simulink model "APP_MyApplication"  (R2018b)
settings: Solver=VariableStepDiscrete  StartTime=0.0  StopTime=10  RelTol=1e-3
PreLoadFcn:
  | if(exist('MBDS_ModelCallback', 'file')), MBDS_ModelCallback('PreLoad'); end;
PostLoadFcn:
  | if(exist('MBDS_ModelCallback', 'file')), MBDS_ModelCallback('PostLoad'); end;
InitFcn:
  | if(exist('MBDS_ModelCallback', 'file')), MBDS_ModelCallback('Init'); end;
StartFcn:
  | if(exist('MBDS_ModelCallback', 'file')), MBDS_ModelCallback('Start'); end;
StopFcn:
  | if(exist('MBDS_ModelCallback', 'file')), MBDS_ModelCallback('Stop'); end;
undefined symbols (not defined in the file): sigbuilder_block, Ts
libraries: KIBES_Signal x499, simulink x8
(part 9 of 10)

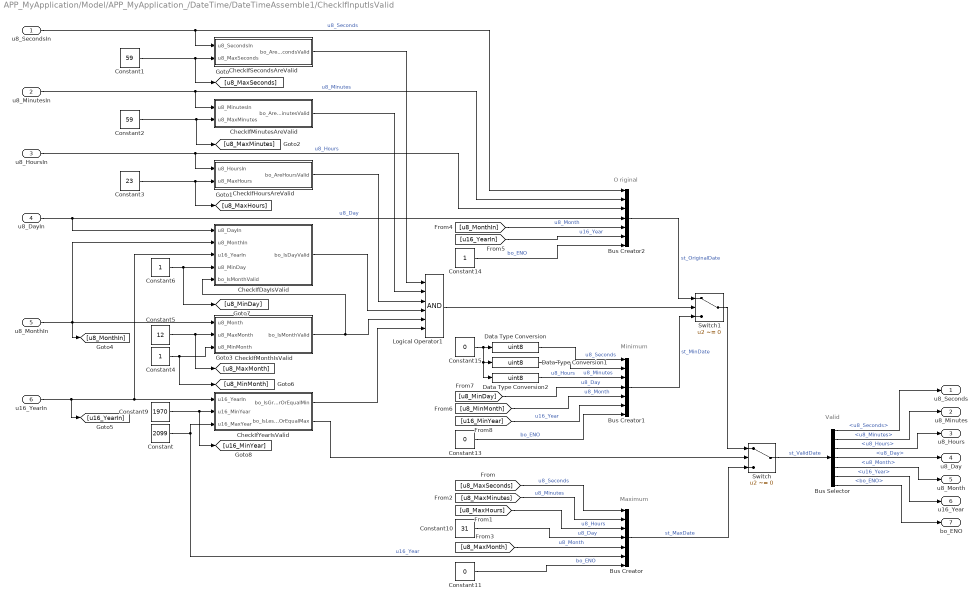
== system APP_MyApplication/Model/APP_MyApplication_/DateTime/DateTimeAssemble1/CheckIfInputIsValid ==
  note: Valid
  note: O riginal
  note: Minimum
  note: Maximum
  u8_SecondsIn : Inport  OutDataTypeStr=uint8
  u8_MinutesIn : Inport  Port=2  OutDataTypeStr=uint8
  u8_HoursIn : Inport  Port=3  OutDataTypeStr=uint8
  u8_DayIn : Inport  Port=4  OutDataTypeStr=uint8
  u8_MonthIn : Inport  Port=5  OutDataTypeStr=uint8
  u16_YearIn : Inport  Port=6  OutDataTypeStr=uint16
  Bus Creator : BusCreator  Inputs='u8_Seconds','u8_Minutes','u8_Hours','u8_Day','u8_Month','u16_Year','bo_ENO'
  Bus Creator1 : BusCreator  Inputs='u8_Seconds','u8_Minutes','u8_Hours','u8_Day','u8_Month','u16_Year','bo_ENO'
  Bus Creator2 : BusCreator  Inputs='u8_Seconds','u8_Minutes','u8_Hours','u8_Day','u8_Month','u16_Year','bo_ENO'
  Bus Selector : BusSelector  OutputSignals=u8_Seconds,u8_Minutes,u8_Hours,u8_Day,u8_Month,u16_Year,bo_ENO
  CheckIfDayIsValid : Subsystem
  CheckIfHoursAreValid : Subsystem
  CheckIfMinutesAreValid : Subsystem
  CheckIfMonthIsValid : Subsystem
  CheckIfSecondsAreValid : Subsystem
  CheckIfYearIsValid : Subsystem
  Constant : Constant  Value=2099  OutDataTypeStr=uint16
  Constant1 : Constant  Value=59  OutDataTypeStr=uint8
  Constant10 : Constant  Value=31  OutDataTypeStr=uint8
  Constant11 : Constant  Value=0  OutDataTypeStr=boolean
  Constant13 : Constant  Value=0  OutDataTypeStr=boolean
  Constant14 : Constant  OutDataTypeStr=boolean
  Constant15 : Constant  Value=0  OutDataTypeStr=uint8
  Constant2 : Constant  Value=59  OutDataTypeStr=uint8
  Constant3 : Constant  Value=23  OutDataTypeStr=uint8
  Constant4 : Constant  OutDataTypeStr=uint8
  Constant5 : Constant  Value=12  OutDataTypeStr=uint8
  Constant6 : Constant  OutDataTypeStr=uint8
  Constant9 : Constant  Value=1970  OutDataTypeStr=uint16
  Data Type Conversion : DataTypeConversion  OutDataTypeStr=uint8
  Data Type Conversion1 : DataTypeConversion  OutDataTypeStr=uint8
  Data Type Conversion2 : DataTypeConversion  OutDataTypeStr=uint8
  Logical Operator1 : Logic  Inputs=6  AllPortsSameDT=off  OutDataTypeStr=boolean
  Switch : Switch  Criteria=u2 ~= 0
  Switch1 : Switch  Criteria=u2 ~= 0
  u8_Seconds : Outport  OutDataTypeStr=uint8
  u8_Minutes : Outport  Port=2  OutDataTypeStr=uint8
  u8_Hours : Outport  Port=3  OutDataTypeStr=uint8
  u8_Day : Outport  Port=4  OutDataTypeStr=uint8
  u8_Month : Outport  Port=5  OutDataTypeStr=uint8
  u16_Year : Outport  Port=6  OutDataTypeStr=uint16
  bo_ENO : Outport  Port=7  OutDataTypeStr=boolean
  wires:
  u16_YearIn/1 -> CheckIfYearIsValid/1(u16_YearIn), CheckIfDayIsValid/3(u16_YearIn), [u16_YearIn]
  Constant/1 -> Bus Creator/6, CheckIfYearIsValid/3(u16_MaxYear)  "u16_Year"
  u8_HoursIn/1 -> Bus Creator2/3, CheckIfHoursAreValid/1(u8_HoursIn)  "u8_Hours"
  u8_MinutesIn/1 -> Bus Creator2/2, CheckIfMinutesAreValid/1(u8_MinutesIn)  "u8_Minutes"
  u8_SecondsIn/1 -> CheckIfSecondsAreValid/1(u8_SecondsIn), Bus Creator2/1  "u8_Seconds"
  u8_DayIn/1 -> Bus Creator2/4, CheckIfDayIsValid/1(u8_DayIn)  "u8_Day"
  Constant5/1 -> CheckIfMonthIsValid/2(u8_MaxMonth), [u8_MaxMonth]
  CheckIfMinutesAreValid/1(bo_AreMinutesValid) -> Logical Operator1/2
  CheckIfHoursAreValid/1(bo_AreHoursValid) -> Logical Operator1/3
  Constant9/1 -> [u16_MinYear], CheckIfYearIsValid/2(u16_MinYear)
  Constant11/1 -> Bus Creator/7  "bo_ENO"
  [u8_MaxMinutes] -> Bus Creator/2  "u8_Minutes"
  [u8_MaxHours] -> Bus Creator/3  "u8_Hours"
  Constant3/1 -> CheckIfHoursAreValid/2(u8_MaxHours), [u8_MaxHours]
  Constant10/1 -> Bus Creator/4  "u8_Day"
  [u8_MaxMonth] -> Bus Creator/5  "u8_Month"
  [u8_MinMonth] -> Bus Creator1/5  "u8_Month"
  Logical Operator1/1 -> Switch1/2
  Bus Creator1/1 -> Switch1/3  "st_MinDate"
  [u8_MonthIn] -> Bus Creator2/5  "u8_Month"
  [u16_YearIn] -> Bus Creator2/6  "u16_Year"
  Constant13/1 -> Bus Creator1/7  "bo_ENO"
  Bus Selector/4 -> u8_Day/1  "<u8_Day>"
  Bus Selector/3 -> u8_Hours/1  "<u8_Hours>"
  Bus Selector/2 -> u8_Minutes/1  "<u8_Minutes>"
  Bus Selector/1 -> u8_Seconds/1  "<u8_Seconds>"
  Bus Selector/6 -> u16_Year/1  "<u16_Year>"
  Bus Selector/7 -> bo_ENO/1  "<bo_ENO>"
  Bus Creator2/1 -> Switch1/1  "st_OriginalDate"
  Switch1/1 -> Switch/1
  Bus Creator/1 -> Switch/3  "st_MaxDate"
  Switch/1 -> Bus Selector/1  "st_ValidDate"
  Constant14/1 -> Bus Creator2/7  "bo_ENO"
  Data Type Conversion/1 -> Bus Creator1/1  "u8_Seconds"
  [u8_MinDay] -> Bus Creator1/4  "u8_Day"
  Constant15/1 -> Data Type Conversion2/1, Data Type Conversion1/1, Data Type Conversion/1
  [u8_MaxSeconds] -> Bus Creator/1  "u8_Seconds"
  Bus Selector/5 -> u8_Month/1  "<u8_Month>"
  u8_MonthIn/1 -> CheckIfDayIsValid/2(u8_MonthIn), [u8_MonthIn], CheckIfMonthIsValid/1(u8_Month)
  CheckIfDayIsValid/1(bo_IsDayValid) -> Logical Operator1/4
  Constant1/1 -> [u8_MaxSeconds], CheckIfSecondsAreValid/2(u8_MaxSeconds)
  CheckIfSecondsAreValid/1(bo_AreSecondsValid) -> Logical Operator1/1
  Constant2/1 -> [u8_MaxMinutes], CheckIfMinutesAreValid/2(u8_MaxMinutes)
  CheckIfMonthIsValid/1(bo_IsMonthValid) -> CheckIfDayIsValid/5(bo_IsMonthValid), Logical Operator1/5
  CheckIfYearIsValid/1(bo_IsGreaterOrEqualMin) -> Logical Operator1/6
  CheckIfYearIsValid/2(bo_IsLessOrEqualMax) -> Switch/2
  Constant4/1 -> [u8_MinMonth], CheckIfMonthIsValid/3(u8_MinMonth)
  Constant6/1 -> [u8_MinDay], CheckIfDayIsValid/4(u8_MinDay)
  [u16_MinYear] -> Bus Creator1/6  "u16_Year"
  Data Type Conversion1/1 -> Bus Creator1/2  "u8_Minutes"
  Data Type Conversion2/1 -> Bus Creator1/3  "u8_Hours"

== system APP_MyApplication/Model/APP_MyApplication_/DateTime/DateTimeAssemble1/ConvertToDateTime ==
  u8_Seconds : Inport  OutDataTypeStr=uint8
  u8_Minutes : Inport  Port=2  OutDataTypeStr=uint8
  u8_Hours : Inport  Port=3  OutDataTypeStr=uint8
  u16_NrOfDays : Inport  Port=4  OutDataTypeStr=uint16
  Add : Sum  Inputs=++++  OutDataTypeStr=uint32
  ConvertDaysToSeconds : Subsystem
  ConvertHoursToSeconds : Subsystem
  ConvertMinutesToSeconds : Subsystem
  u32_DateTime : Outport  OutDataTypeStr=uint32
  wires:
  u8_Seconds/1 -> Add/1
  Add/1 -> u32_DateTime/1
  ConvertMinutesToSeconds/1(u16_SecFromMins) -> Add/2
  ConvertHoursToSeconds/1(u32_SecFromHrs) -> Add/3
  ConvertDaysToSeconds/1(u32_SecFromDays) -> Add/4
  u8_Minutes/1 -> ConvertMinutesToSeconds/1(u8_Minutes)
  u8_Hours/1 -> ConvertHoursToSeconds/1(u8_Hours)
  u16_NrOfDays/1 -> ConvertDaysToSeconds/1(u16_NrOfDays)

== system APP_MyApplication/Model/APP_MyApplication_/DateTime/DateTimeAssemble1/ConvertToNrOfDays ==
  note: Convert to number of days
  u8_Day : Inport  OutDataTypeStr=uint8
  u8_Month : Inport  Port=2  OutDataTypeStr=uint8
  u16_Year : Inport  Port=3  OutDataTypeStr=uint16
  AddDays : Subsystem
  AddDaysForCompleteMonths : Subsystem  TreatAsAtomicUnit=on
  AddDaysForCompleteYears : Subsystem
  CheckIfDateInLeapYearBeforeMarch : Subsystem
  Subtract2 : Sum  Inputs=+++-  OutDataTypeStr=uint16
  u16_NrOfDays : Outport  OutDataTypeStr=uint16
  wires:
  u16_Year/1 -> CheckIfDateInLeapYearBeforeMarch/2(u16_Year), AddDaysForCompleteYears/1(u16_Year)
  Subtract2/1 -> u16_NrOfDays/1
  u8_Month/1 -> CheckIfDateInLeapYearBeforeMarch/1(u8_Month), AddDaysForCompleteMonths/1(u8_Month)
  u8_Day/1 -> AddDays/1(u8_Day)
  AddDaysForCompleteMonths/1(u16_DaysForMonths) -> Subtract2/2
  AddDays/1(u8_CompleteDays) -> Subtract2/1
  AddDaysForCompleteYears/1(u16_DaysForYears) -> Subtract2/3
  CheckIfDateInLeapYearBeforeMarch/1(bo_MinusOne) -> Subtract2/4

== system APP_MyApplication/Model/APP_MyApplication_/DateTime/DateTimeDisassemble/CheckIfTimeDataIsValid ==
  note: 2099-12-31-23:59:59
  note: Check if time data is valid
  u32_DateTime : Inport  OutDataTypeStr=uint32
  Constant14 : Constant  Value=4102444799  OutDataTypeStr=uint32
  Relational Operator : RelationalOperator  Operator=<=  OutDataTypeStr=boolean  RndMeth=Nearest
  bo_ENO : Outport  OutDataTypeStr=boolean
  wires:
  Constant14/1 -> Relational Operator/2
  u32_DateTime/1 -> Relational Operator/1
  Relational Operator/1 -> bo_ENO/1

== system APP_MyApplication/Model/APP_MyApplication_/DateTime/DateTimeDisassemble/CheckLeapYearsAndRemainingDays ==
  note: Year
  note: Check leap year and calculate remaining days in current year
  note: avoid overflow
  u16_NrOfDays : Inport  OutDataTypeStr=uint16
  Add3 : Sum  Inputs=++-  OutDataTypeStr=uint16
  CalculateLeapYearsSince1970 : Subsystem
  CalculateRemainingDays : Subsystem
  CheckIfCorrectedTempYearIsLeap : Subsystem
  CheckIfTempYearIsCorrect : Subsystem
  CheckLeapYear : Subsystem
  Constant2 : Constant  OutDataTypeStr=uint16
  Constant6 : Constant  Value=0  OutDataTypeStr=uint16
  DaysPerNonLeapYear : Constant  Value=365  OutDataTypeStr=uint16
  Math Function3 : Math  Operator=rem  OutputSignalType=real  SaturateOnIntegerOverflow=on
  Relational Operator1 : RelationalOperator  Operator===  OutDataTypeStr=boolean  RndMeth=Nearest  InputSameDT=on
  Switch1 : Switch  Criteria=u2 ~= 0  OutDataTypeStr=uint16
  u16_TempDate : Outport  OutDataTypeStr=uint16
  u16_Year : Outport  Port=2  OutDataTypeStr=uint16
  bo_LeapYear : Outport  Port=3  OutDataTypeStr=boolean
  wires:
  u16_NrOfDays/1 -> CalculateLeapYearsSince1970/1(u16_NrOfDays), Math Function3/1
  DaysPerNonLeapYear/1 -> CalculateRemainingDays/5(u16_DaysPerCommonYear), Math Function3/2, CalculateLeapYearsSince1970/2(u16_DaysPerCommonYear)
  Math Function3/1 -> CalculateRemainingDays/3(u16_TempRemainingDays), CheckIfTempYearIsCorrect/1(u16_TempRemainingDays)
  Switch1/1 -> CheckLeapYear/1(u16_Year), u16_Year/1
  CalculateLeapYearsSince1970/2(u16_TempYear) -> Switch1/1, Add3/2, Relational Operator1/2
  Add3/1 -> Switch1/3, CheckIfCorrectedTempYearIsLeap/1(u16_CorrectedTempYear)
  CheckLeapYear/1(bo_LeapYear) -> bo_LeapYear/1
  Constant6/1 -> Relational Operator1/1
  Constant2/1 -> Add3/3
  Relational Operator1/1 -> Add3/1
  CalculateLeapYearsSince1970/1(u16_NrOfLeapYears) -> [u16_NrOfLeapYears]
  [u16_NrOfLeapYears] -> CheckIfTempYearIsCorrect/2(u16_NrOfLeapYears)
  CheckIfTempYearIsCorrect/1(bo_IsTempYearCorrect) -> Switch1/2, CalculateRemainingDays/2(bo_IsTempYearCorrect)
  CalculateRemainingDays/1(u16_TempDate) -> u16_TempDate/1
  CheckIfCorrectedTempYearIsLeap/1(bo_IsCorrectedYearLeapYear) -> CalculateRemainingDays/1(bo_IsCorrectedYearLeapYear)
  [u16_NrOfLeapYears] -> CalculateRemainingDays/4(u16_NrOfLeapYears)

== system APP_MyApplication/Model/APP_MyApplication_/DateTime/DateTimeDisassemble/ConvertToDayOfWeek ==
  note: 1970-01-01 is Thursday
  note: Convert to day of week
  u16_NrOfDays : Inport  OutDataTypeStr=uint16
  Add2 : Sum  OutDataTypeStr=uint16
  Add3 : Sum  OutDataTypeStr=uint16
  Constant3 : Constant  Value=7  OutDataTypeStr=uint16
  Constant4 : Constant  Value=3  OutDataTypeStr=uint8
  Constant5 : Constant  OutDataTypeStr=uint8
  Data Type Conversion3 : DataTypeConversion  OutDataTypeStr=uint8
  Math Function : Math  Operator=rem  OutputSignalType=real  SaturateOnIntegerOverflow=on
  u8_DayOfWeek : Outport  OutDataTypeStr=uint8
  wires:
  Data Type Conversion3/1 -> u8_DayOfWeek/1
  Constant5/1 -> Add3/2
  Constant3/1 -> Math Function/2
  Constant4/1 -> Add2/2
  Add2/1 -> Math Function/1
  Math Function/1 -> Add3/1
  Add3/1 -> Data Type Conversion3/1
  u16_NrOfDays/1 -> Add2/1

== system APP_MyApplication/Model/APP_MyApplication_/DateTime/DateTimeDisassemble/ConvertToMonthAndDay ==
  note: Days per month
  note: Count number of cycles (= Month - 1)
  note: Check if there are less days remaining than the next month has
  note: Convert to month and day
  u16_TempDate : Inport  OutDataTypeStr=uint16
  bo_LeapYear : Inport  Port=2  OutDataTypeStr=boolean
  Add5 : Sum  OutDataTypeStr=uint8
  CheckNrOfDaysInNextMonth : Subsystem
  Constant1 : Constant  Value=[0 31 28 31 30 31 30 31 31 30 31 30 31]  OutDataTypeStr=uint8
  Data Type Conversion : DataTypeConversion  OutDataTypeStr=uint8
  Data Type Conversion1 : DataTypeConversion  OutDataTypeStr=uint16
  Relational Operator1 : RelationalOperator  OutDataTypeStr=boolean  RndMeth=Nearest  InputSameDT=on
  SubstractDaysOfMonths : Subsystem
  Unit Delay1 : UnitDelay  SampleTime=-1
  While Iterator : WhileIterator  MaxIters=12  WhileBlockType=do-while  ResetStates=reset  ShowIterationPort=on  OutputDataType=int8
  u8_MonthMinusOne : Outport  OutDataTypeStr=uint8
  u16_DayMinusOne : Outport  Port=2  OutDataTypeStr=uint16
  wires:
  bo_LeapYear/1 -> SubstractDaysOfMonths/2(bo_LeapYear), CheckNrOfDaysInNextMonth/3(bo_LeapYear)
  Relational Operator1/1 -> Data Type Conversion/1, While Iterator/1
  While Iterator/1 -> SubstractDaysOfMonths/3(i8_IterationNr), CheckNrOfDaysInNextMonth/2(i8_IterationNr)
  Add5/1 -> u8_MonthMinusOne/1, Unit Delay1/1
  Unit Delay1/1 -> Add5/2
  Data Type Conversion/1 -> Add5/1
  SubstractDaysOfMonths/1(u16_RemainingDays) -> u16_DayMinusOne/1, Relational Operator1/1
  CheckNrOfDaysInNextMonth/1(u8_DaysInNextMonth) -> Data Type Conversion1/1
  u16_TempDate/1 -> SubstractDaysOfMonths/1(u16_TempDate)
  Constant1/1 -> SubstractDaysOfMonths/4(u8_DaysPerMonth), CheckNrOfDaysInNextMonth/1(u8_DaysPerMonth)
  Data Type Conversion1/1 -> Relational Operator1/2

== system APP_MyApplication/Model/APP_MyApplication_/DateTime/DateTimeDisassemble/ConvertToTimeAndNrOfDays ==
  note: Convert date time to time and number of days
  u32_DateTime : Inport  OutDataTypeStr=uint32
  CalculateHours : Subsystem
  CalculateMinutes : Subsystem
  CalculateSeconds : Subsystem
  u8_Seconds : Outport  OutDataTypeStr=uint8
  u8_Minutes : Outport  Port=2  OutDataTypeStr=uint8
  u8_Hours : Outport  Port=3  OutDataTypeStr=uint8
  u16_NrOfDays : Outport  Port=4  OutDataTypeStr=uint16
  wires:
  CalculateSeconds/1(u8_Seconds) -> u8_Seconds/1
  CalculateHours/2(u16_NrOfDays) -> u16_NrOfDays/1
  u32_DateTime/1 -> CalculateSeconds/1(u32_TimeInSeconds)
  CalculateSeconds/2(u32_TempDateMin) -> CalculateMinutes/1(u32_TempDateMin)
  CalculateMinutes/1(u8_Minutes) -> u8_Minutes/1
  CalculateMinutes/2(u32_TempDateHrs) -> CalculateHours/1(u32_TempDateHrs)
  CalculateHours/1(u8_Hours) -> u8_Hours/1

== system APP_MyApplication/Model/APP_MyApplication_/EEProm/TimerPulse/EdgeRising ==
  note: EdgeRising
  u : Inport  OutDataTypeStr=boolean
  Data Type Duplicate : DataTypeDuplicate
  IV : Constant  Value=0  OutDataTypeStr=Inherit: Inherit via back propagation
  NoReset : Subsystem
  R : Constant  Value=0  OutDataTypeStr=boolean
  Relational Operator : RelationalOperator  Operator=<  OutDataTypeStr=boolean  RndMeth=Nearest  InputSameDT=on
  Unit Delay : UnitDelay  SampleTime=-1
  y : Outport
  wires:
  IV/1 -> NoReset/1(Unused1), Data Type Duplicate/2
  u/1 -> Unit Delay/1, Relational Operator/2, Data Type Duplicate/1
  R/1 -> NoReset/2(Unused2)
  NoReset/1(y) -> Relational Operator/1
  Unit Delay/1 -> NoReset/3(u)
  Relational Operator/1 -> y/1

== system APP_MyApplication/Model/APP_MyApplication_/EEProm/TimerPulse/TimeSource ==
  note: TimeSource
  Constant : Constant  Value=Value  OutDataTypeStr=uint32  LockScale=on
  Out : Outport
  wires:
  Constant/1 -> Out/1

== system APP_MyApplication/Model/APP_MyApplication_/EEProm/TimerPulse/Timer_RE1 ==
  note: Timer_RE
  R : Inport  OutDataTypeStr=boolean
  IV : Inport  Port=2
  Constant : Constant  Value=0  OutDataTypeStr=Inherit: Inherit via back propagation
  Constant1 : Constant  Value=0  OutDataTypeStr=Inherit: Inherit via back propagation
  Constant2 : Constant  Value=0  OutDataTypeStr=Inherit: Inherit via back propagation
  Data Type Duplicate : DataTypeDuplicate  NumInputPorts=3
  DoubleReset : Subsystem
  E : Constant  OutDataTypeStr=boolean
  NoEnable : Subsystem
  Relational Operator : RelationalOperator  Operator=<=  OutDataTypeStr=boolean  RndMeth=Nearest
  Relational Operator1 : RelationalOperator  Operator=>  OutDataTypeStr=boolean  RndMeth=Nearest
  Relational Operator2 : RelationalOperator  Operator=>  OutDataTypeStr=boolean  RndMeth=Nearest  InputSameDT=on
  Subtract : Sum  Inputs=+-  OutDataTypeStr=Inherit: Inherit via back propagation
  Switch1 : Switch  Criteria=u2 ~= 0  OutDataTypeStr=Inherit: Inherit via back propagation
  Unit Delay : UnitDelay  SampleTime=-1
  dT : Constant  Value=1000*Ts  OutDataTypeStr=Inherit: Inherit via back propagation
  x : Terminator
  y : Outport
  wires:
  R/1 -> DoubleReset/2(R1)
  E/1 -> NoEnable/2(Unused1)
  IV/1 -> Data Type Duplicate/1, DoubleReset/1(IV)
  Relational Operator/1 -> DoubleReset/3(R2)
  DoubleReset/1(y) -> Relational Operator2/1, Unit Delay/1, x/1, Data Type Duplicate/3
  Constant2/1 -> Relational Operator2/2
  Constant/1 -> Switch1/3
  Subtract/1 -> Switch1/1
  Relational Operator1/1 -> Switch1/2
  Switch1/1 -> NoEnable/1(u)
  dT/1 -> Subtract/2, Relational Operator1/2
  Unit Delay/1 -> NoEnable/3(Unused2), Relational Operator1/1, Subtract/1, Relational Operator/1, Data Type Duplicate/2
  Constant1/1 -> Relational Operator/2
  NoEnable/1(y) -> DoubleReset/4(u)
  Relational Operator2/1 -> y/1

== system APP_MyApplication/Model/APP_MyApplication_/EEProm/TimerPulse1/EdgeRising ==
  note: EdgeRising
  u : Inport  OutDataTypeStr=boolean
  Data Type Duplicate : DataTypeDuplicate
  IV : Constant  Value=0  OutDataTypeStr=Inherit: Inherit via back propagation
  NoReset : Subsystem
  R : Constant  Value=0  OutDataTypeStr=boolean
  Relational Operator : RelationalOperator  Operator=<  OutDataTypeStr=boolean  RndMeth=Nearest  InputSameDT=on
  Unit Delay : UnitDelay  SampleTime=-1
  y : Outport
  wires:
  IV/1 -> NoReset/1(Unused1), Data Type Duplicate/2
  u/1 -> Unit Delay/1, Relational Operator/2, Data Type Duplicate/1
  R/1 -> NoReset/2(Unused2)
  NoReset/1(y) -> Relational Operator/1
  Unit Delay/1 -> NoReset/3(u)
  Relational Operator/1 -> y/1

== system APP_MyApplication/Model/APP_MyApplication_/EEProm/TimerPulse1/TimeSource ==
  note: TimeSource
  Constant : Constant  Value=Value  OutDataTypeStr=uint32  LockScale=on
  Out : Outport
  wires:
  Constant/1 -> Out/1

== system APP_MyApplication/Model/APP_MyApplication_/EEProm/TimerPulse1/Timer_RE1 ==
  note: Timer_RE
  R : Inport  OutDataTypeStr=boolean
  IV : Inport  Port=2
  Constant : Constant  Value=0  OutDataTypeStr=Inherit: Inherit via back propagation
  Constant1 : Constant  Value=0  OutDataTypeStr=Inherit: Inherit via back propagation
  Constant2 : Constant  Value=0  OutDataTypeStr=Inherit: Inherit via back propagation
  Data Type Duplicate : DataTypeDuplicate  NumInputPorts=3
  DoubleReset : Subsystem
  E : Constant  OutDataTypeStr=boolean
  NoEnable : Subsystem
  Relational Operator : RelationalOperator  Operator=<=  OutDataTypeStr=boolean  RndMeth=Nearest
  Relational Operator1 : RelationalOperator  Operator=>  OutDataTypeStr=boolean  RndMeth=Nearest
  Relational Operator2 : RelationalOperator  Operator=>  OutDataTypeStr=boolean  RndMeth=Nearest  InputSameDT=on
  Subtract : Sum  Inputs=+-  OutDataTypeStr=Inherit: Inherit via back propagation
  Switch1 : Switch  Criteria=u2 ~= 0  OutDataTypeStr=Inherit: Inherit via back propagation
  Unit Delay : UnitDelay  SampleTime=-1
  dT : Constant  Value=1000*Ts  OutDataTypeStr=Inherit: Inherit via back propagation
  x : Terminator
  y : Outport
  wires:
  R/1 -> DoubleReset/2(R1)
  E/1 -> NoEnable/2(Unused1)
  IV/1 -> Data Type Duplicate/1, DoubleReset/1(IV)
  Relational Operator/1 -> DoubleReset/3(R2)
  DoubleReset/1(y) -> Relational Operator2/1, Unit Delay/1, x/1, Data Type Duplicate/3
  Constant2/1 -> Relational Operator2/2
  Constant/1 -> Switch1/3
  Subtract/1 -> Switch1/1
  Relational Operator1/1 -> Switch1/2
  Switch1/1 -> NoEnable/1(u)
  dT/1 -> Subtract/2, Relational Operator1/2
  Unit Delay/1 -> NoEnable/3(Unused2), Relational Operator1/1, Subtract/1, Relational Operator/1, Data Type Duplicate/2
  Constant1/1 -> Relational Operator/2
  NoEnable/1(y) -> DoubleReset/4(u)
  Relational Operator2/1 -> y/1

== system APP_MyApplication/Model/APP_MyApplication_/TimerPulse/EdgeRising/NoReset ==
  Unused1 : Inport
  Unused2 : Inport  Port=2
  u : Inport  Port=3
  Terminator : Terminator
  Terminator1 : Terminator
  y : Outport
  wires:
  u/1 -> y/1
  Unused1/1 -> Terminator1/1
  Unused2/1 -> Terminator/1

== system APP_MyApplication/Model/APP_MyApplication_/TimerPulse/Timer_RE1/DoubleReset ==
  IV : Inport
  R1 : Inport  Port=2
  R2 : Inport  Port=3
  u : Inport  Port=4
  Logical Operator : Logic  AllPortsSameDT=off  OutDataTypeStr=boolean
  Switch1 : Switch  Criteria=u2 ~= 0  OutDataTypeStr=Inherit: Inherit via back propagation  InputSameDT=on
  y : Outport
  wires:
  u/1 -> Switch1/3
  Switch1/1 -> y/1
  IV/1 -> Switch1/1
  Logical Operator/1 -> Switch1/2
  R1/1 -> Logical Operator/1
  R2/1 -> Logical Operator/2

== system APP_MyApplication/Model/APP_MyApplication_/TimerPulse/Timer_RE1/NoEnable ==
  u : Inport
  Unused1 : Inport  Port=2
  Unused2 : Inport  Port=3
  Terminator : Terminator
  Terminator1 : Terminator
  y : Outport
  wires:
  Unused2/1 -> Terminator1/1
  u/1 -> y/1
  Unused1/1 -> Terminator/1

== system APP_MyApplication/Model/APP_MyApplication_/DTC/DateTimeDisassemble/CheckLeapYearsAndRemainingDays/CalculateLeapYearsSince1970 ==
  u16_NrOfDays : Inport  OutDataTypeStr=uint16
  u16_DaysPerCommonYear : Inport  Port=2  OutDataTypeStr=uint16
  Add : Sum  OutDataTypeStr=uint16
  Constant : Constant  OutDataTypeStr=uint16
  Constant1 : Constant  Value=4  OutDataTypeStr=uint16
  Divide : Product  Inputs=*/  OutDataTypeStr=uint16
  Divide1 : Product  Inputs=*/  OutDataTypeStr=uint16
  u16_NrOfLeapYears : Outport  OutDataTypeStr=uint16
  u16_TempYear : Outport  Port=2  OutDataTypeStr=uint16
  wires:
  Divide/1 -> Add/1, u16_TempYear/1
  Constant/1 -> Add/2
  Constant1/1 -> Divide1/2
  Add/1 -> Divide1/1
  Divide1/1 -> u16_NrOfLeapYears/1
  u16_NrOfDays/1 -> Divide/1
  u16_DaysPerCommonYear/1 -> Divide/2

== system APP_MyApplication/Model/APP_MyApplication_/DTC/DateTimeDisassemble/CheckLeapYearsAndRemainingDays/CalculateRemainingDays ==
  bo_IsCorrectedYearLeapYear : Inport  OutDataTypeStr=boolean
  bo_IsTempYearCorrect : Inport  Port=2  OutDataTypeStr=boolean
  u16_TempRemainingDays : Inport  Port=3  OutDataTypeStr=uint16
  u16_NrOfLeapYears : Inport  Port=4  OutDataTypeStr=uint16
  u16_DaysPerCommonYear : Inport  Port=5  OutDataTypeStr=uint16
  Add : Sum  OutDataTypeStr=uint16
  Add1 : Sum  Inputs=++-  OutDataTypeStr=uint16
  Constant : Constant  OutDataTypeStr=uint16
  Subtract : Sum  Inputs=+-  OutDataTypeStr=uint16  SaturateOnIntegerOverflow=on
      settings: AttributesFormatString=Saturate: %<SaturateOnIntegerOverflow>
  Switch : Switch  Criteria=u2 ~= 0  OutDataTypeStr=uint16
  Switch1 : Switch  Criteria=u2 ~= 0  OutDataTypeStr=uint16
  u16_TempDate : Outport  OutDataTypeStr=uint16
  wires:
  u16_TempRemainingDays/1 -> Add1/1, Subtract/1
  u16_NrOfLeapYears/1 -> Add1/3, Subtract/2
  u16_DaysPerCommonYear/1 -> Add1/2
  Constant/1 -> Add/1
  bo_IsCorrectedYearLeapYear/1 -> Switch1/2
  Add1/1 -> Add/2, Switch1/3
  Add/1 -> Switch1/1
  Switch1/1 -> Switch/3
  Switch/1 -> u16_TempDate/1
  bo_IsTempYearCorrect/1 -> Switch/2
  Subtract/1 -> Switch/1

== system APP_MyApplication/Model/APP_MyApplication_/DTC/DateTimeDisassemble/CheckLeapYearsAndRemainingDays/CheckIfCorrectedTempYearIsLeap ==
  u16_CorrectedTempYear : Inport  OutDataTypeStr=uint16
  Add : Sum  OutDataTypeStr=uint16
  Constant : Constant  Value=2  OutDataTypeStr=uint16
  Constant1 : Constant  Value=4  OutDataTypeStr=uint16
  Constant2 : Constant  Value=0  OutDataTypeStr=uint16
  Math Function : Math  Operator=rem  OutputSignalType=real  SaturateOnIntegerOverflow=on
  Relational Operator : RelationalOperator  Operator===  OutDataTypeStr=boolean  RndMeth=Nearest
  bo_IsCorrectedYearLeapYear : Outport  OutDataTypeStr=boolean
  wires:
  u16_CorrectedTempYear/1 -> Add/1
  Add/1 -> Math Function/1
  Math Function/1 -> Relational Operator/1
  Constant/1 -> Add/2
  Constant1/1 -> Math Function/2
  Constant2/1 -> Relational Operator/2
  Relational Operator/1 -> bo_IsCorrectedYearLeapYear/1

== system APP_MyApplication/Model/APP_MyApplication_/DTC/DateTimeDisassemble/CheckLeapYearsAndRemainingDays/CheckIfTempYearIsCorrect ==
  u16_TempRemainingDays : Inport  OutDataTypeStr=uint16
  u16_NrOfLeapYears : Inport  Port=2  OutDataTypeStr=uint16
  Relational Operator : RelationalOperator  OutDataTypeStr=boolean  RndMeth=Nearest
  bo_IsTempYearCorrect : Outport  OutDataTypeStr=boolean
  wires:
  u16_TempRemainingDays/1 -> Relational Operator/1
  u16_NrOfLeapYears/1 -> Relational Operator/2
  Relational Operator/1 -> bo_IsTempYearCorrect/1

== system APP_MyApplication/Model/APP_MyApplication_/DTC/DateTimeDisassemble/CheckLeapYearsAndRemainingDays/CheckLeapYear ==
  note: check if the current year is a leap year
  u16_Year : Inport  OutDataTypeStr=uint16
  Add6 : Sum  OutDataTypeStr=uint16
  Constant : Constant  Value=2  OutDataTypeStr=uint8
  Constant1 : Constant  Value=4  OutDataTypeStr=uint16
  Constant9 : Constant  Value=0  OutDataTypeStr=uint16
  Math Function : Math  Operator=rem  OutputSignalType=real  SaturateOnIntegerOverflow=on
  Relational Operator2 : RelationalOperator  Operator===  OutDataTypeStr=boolean  RndMeth=Nearest  InputSameDT=on
  bo_LeapYear : Outport  OutDataTypeStr=boolean
  wires:
  Add6/1 -> Math Function/1
  Relational Operator2/1 -> bo_LeapYear/1
  u16_Year/1 -> Add6/1
  Math Function/1 -> Relational Operator2/1
  Constant9/1 -> Relational Operator2/2
  Constant/1 -> Add6/2
  Constant1/1 -> Math Function/2

== system APP_MyApplication/Model/APP_MyApplication_/DTC/DateTimeDisassemble/ConvertToMonthAndDay/CheckNrOfDaysInNextMonth ==
  u8_DaysPerMonth : Inport  OutDataTypeStr=uint8
  i8_IterationNr : Inport  Port=2  OutDataTypeStr=int8
  bo_LeapYear : Inport  Port=3  OutDataTypeStr=boolean
  Add1 : Sum  OutDataTypeStr=uint8
  CheckNextMonthFebLeapYear : Subsystem
  Selector : Selector  IndexMode=Zero-based  InputPortWidth=13  IndexOptions=Index vector (port)  Indices=[1 3]  OutputSizes=1
  u8_DaysInNextMonth : Outport  OutDataTypeStr=uint8
  wires:
  bo_LeapYear/1 -> CheckNextMonthFebLeapYear/2(bo_LeapYear)
  i8_IterationNr/1 -> Selector/2, CheckNextMonthFebLeapYear/1(i8_IterationNr)
  u8_DaysPerMonth/1 -> Selector/1
  Selector/1 -> Add1/1
  CheckNextMonthFebLeapYear/1(bo_IsNextFebLeapYear) -> Add1/2
  Add1/1 -> u8_DaysInNextMonth/1

== system APP_MyApplication/Model/APP_MyApplication_/DTC/DateTimeDisassemble/ConvertToMonthAndDay/SubstractDaysOfMonths ==
  u16_TempDate : Inport  OutDataTypeStr=uint16
  bo_LeapYear : Inport  Port=2  OutDataTypeStr=boolean
  i8_IterationNr : Inport  Port=3  OutDataTypeStr=int8
  u8_DaysPerMonth : Inport  Port=4  OutDataTypeStr=uint8
  Add : Sum  OutDataTypeStr=uint16
  Add1 : Sum  OutDataTypeStr=uint16
  Add2 : Sum  Inputs=+-  OutDataTypeStr=uint8
  CheckCurrMonthFebLeapYear : Subsystem
  Constant : Constant  OutDataTypeStr=int8
  Selector : Selector  IndexMode=Zero-based  InputPortWidth=13  IndexOptions=Index vector (port)  Indices=[1 3]  OutputSizes=1
  Subtract : Sum  Inputs=+-  OutDataTypeStr=uint16
  Unit Delay : UnitDelay  SampleTime=-1
  u16_RemainingDays : Outport  OutDataTypeStr=uint16
  wires:
  bo_LeapYear/1 -> CheckCurrMonthFebLeapYear/1(bo_LeapYear)
  i8_IterationNr/1 -> Add2/1, CheckCurrMonthFebLeapYear/2(i8_IterationNr)
  u8_DaysPerMonth/1 -> Selector/1
  u16_TempDate/1 -> Subtract/1
  Subtract/1 -> u16_RemainingDays/1
  CheckCurrMonthFebLeapYear/1(bo_IsCurrFebLeapYear) -> Add/1
  Selector/1 -> Add/2
  Add/1 -> Add1/1
  Add1/1 -> Subtract/2, Unit Delay/1
  Unit Delay/1 -> Add1/2
  Add2/1 -> Selector/2
  Constant/1 -> Add2/2

== system APP_MyApplication/Model/APP_MyApplication_/DTC/DateTimeDisassemble/ConvertToTimeAndNrOfDays/CalculateHours ==
  note: 24 hrs/d
  u32_TempDateHrs : Inport  OutDataTypeStr=uint32
  Constant : Constant  Value=24  OutDataTypeStr=uint32
  Data Type Conversion : DataTypeConversion  OutDataTypeStr=uint8
  Data Type Conversion1 : DataTypeConversion  OutDataTypeStr=uint16
  Divide : Product  Inputs=*/  OutDataTypeStr=uint32
  Math Function : Math  Operator=rem  OutputSignalType=real  SaturateOnIntegerOverflow=on
  u8_Hours : Outport  OutDataTypeStr=uint8
  u16_NrOfDays : Outport  Port=2  OutDataTypeStr=uint16
  wires:
  Math Function/1 -> Data Type Conversion/1
  Data Type Conversion/1 -> u8_Hours/1
  Divide/1 -> Data Type Conversion1/1
  Data Type Conversion1/1 -> u16_NrOfDays/1
  Constant/1 -> Math Function/2, Divide/2
  u32_TempDateHrs/1 -> Divide/1, Math Function/1

== system APP_MyApplication/Model/APP_MyApplication_/DTC/DateTimeDisassemble/ConvertToTimeAndNrOfDays/CalculateMinutes ==
  note: 60 min/h
  u32_TempDateMin : Inport  OutDataTypeStr=uint32
  Constant1 : Constant  Value=60  OutDataTypeStr=uint32
  Data Type Conversion1 : DataTypeConversion  OutDataTypeStr=uint8
  Divide : Product  Inputs=*/  OutDataTypeStr=uint32
  Math Function : Math  Operator=rem  OutputSignalType=real  SaturateOnIntegerOverflow=on
  u8_Minutes : Outport  OutDataTypeStr=uint8
  u32_TempDateHrs : Outport  Port=2  OutDataTypeStr=uint32
  wires:
  Math Function/1 -> Data Type Conversion1/1
  u32_TempDateMin/1 -> Divide/1, Math Function/1
  Divide/1 -> u32_TempDateHrs/1
  Constant1/1 -> Math Function/2, Divide/2
  Data Type Conversion1/1 -> u8_Minutes/1

== system APP_MyApplication/Model/APP_MyApplication_/DTC/DateTimeDisassemble/ConvertToTimeAndNrOfDays/CalculateSeconds ==
  note: 60 sec/min
  u32_TimeInSeconds : Inport  OutDataTypeStr=uint32
  Constant : Constant  Value=60  OutDataTypeStr=uint32
  Data Type Conversion : DataTypeConversion  OutDataTypeStr=uint8
  Divide : Product  Inputs=*/  OutDataTypeStr=uint32
  Math Function : Math  Operator=rem  OutputSignalType=real  SaturateOnIntegerOverflow=on
  u8_Seconds : Outport  OutDataTypeStr=uint8
  u32_TempDateMin : Outport  Port=2  OutDataTypeStr=uint32
  wires:
  u32_TimeInSeconds/1 -> Divide/1, Math Function/1
  Math Function/1 -> Data Type Conversion/1
  Data Type Conversion/1 -> u8_Seconds/1
  Constant/1 -> Divide/2, Math Function/2
  Divide/1 -> u32_TempDateMin/1

== system APP_MyApplication/Model/APP_MyApplication_/DateTime/DateTimeAssemble/CheckIfInputIsValid/CheckIfDayIsValid ==
  note: Index correction
  note: days per month
  note: check if day data is valid
  u8_DayIn : Inport  OutDataTypeStr=uint8
  u8_MonthIn : Inport  Port=2  OutDataTypeStr=uint8
  u16_YearIn : Inport  Port=3  OutDataTypeStr=uint16
  u8_MinDay : Inport  Port=4  OutDataTypeStr=uint8
  bo_IsMonthValid : Inport  Port=5  OutDataTypeStr=boolean
  CheckIfFebruaryOfLeapYear : Subsystem
  Constant1 : Constant  OutDataTypeStr=uint8
  Constant2 : Constant  Value=[31 28 31 30 31 30 31 31 30 31 30 31]  OutDataTypeStr=uint8
  Constant20 : Constant  OutDataTypeStr=uint8
  Logical Operator1 : Logic  AllPortsSameDT=off  OutDataTypeStr=boolean
  Logical Operator3 : Logic  Operator=OR  AllPortsSameDT=off  OutDataTypeStr=boolean
  Relational Operator4 : RelationalOperator  Operator=<=  OutDataTypeStr=boolean  RndMeth=Nearest
  Relational Operator8 : RelationalOperator  OutDataTypeStr=boolean  RndMeth=Nearest
  Selector : Selector  IndexMode=Zero-based  InputPortWidth=12  IndexOptions=Index vector (port)  Indices=[1 3]  OutputSizes=1
  Subtract : Sum  Inputs=+-  OutDataTypeStr=uint8
      settings: AttributesFormatString=Saturate: %<SaturateOnIntegerOverflow>
  Switch2 : Switch  Criteria=u2 > Threshold  OutDataTypeStr=uint8
  bo_IsDayValid : Outport  OutDataTypeStr=boolean
  wires:
  u16_YearIn/1 -> CheckIfFebruaryOfLeapYear/3(u16_YearIn)
  Constant2/1 -> Selector/1
  u8_MonthIn/1 -> CheckIfFebruaryOfLeapYear/2(u8_MonthIn), Switch2/1
  Selector/1 -> Relational Operator4/2
  Relational Operator4/1 -> Logical Operator3/1
  Relational Operator8/1 -> Logical Operator1/1
  Constant20/1 -> Switch2/3
  Logical Operator3/1 -> Logical Operator1/2
  Logical Operator1/1 -> bo_IsDayValid/1
  u8_DayIn/1 -> Relational Operator8/1, Relational Operator4/1, CheckIfFebruaryOfLeapYear/1(u8_DayIn)
  CheckIfFebruaryOfLeapYear/1(bo_IsFebrauryOfLeapYear) -> Logical Operator3/2
  u8_MinDay/1 -> Relational Operator8/2
  bo_IsMonthValid/1 -> Switch2/2
  Switch2/1 -> Subtract/1
  Subtract/1 -> Selector/2
  Constant1/1 -> Subtract/2

== system APP_MyApplication/Model/APP_MyApplication_/DateTime/DateTimeAssemble/CheckIfInputIsValid/CheckIfHoursAreValid ==
  note: check if hours data is valid
  u8_HoursIn : Inport  OutDataTypeStr=uint8
  u8_MaxHours : Inport  Port=2  OutDataTypeStr=uint8
  Relational Operator3 : RelationalOperator  Operator=<=  OutDataTypeStr=boolean  RndMeth=Nearest
  bo_AreHoursValid : Outport  OutDataTypeStr=boolean
  wires:
  Relational Operator3/1 -> bo_AreHoursValid/1
  u8_HoursIn/1 -> Relational Operator3/1
  u8_MaxHours/1 -> Relational Operator3/2

== system APP_MyApplication/Model/APP_MyApplication_/DateTime/DateTimeAssemble/CheckIfInputIsValid/CheckIfMinutesAreValid ==
  note: check if minutes data is valid
  u8_MinutesIn : Inport  OutDataTypeStr=uint8
  u8_MaxMinutes : Inport  Port=2  OutDataTypeStr=uint8
  Relational Operator2 : RelationalOperator  Operator=<=  OutDataTypeStr=boolean  RndMeth=Nearest
  bo_AreMinutesValid : Outport  OutDataTypeStr=boolean
  wires:
  Relational Operator2/1 -> bo_AreMinutesValid/1
  u8_MinutesIn/1 -> Relational Operator2/1
  u8_MaxMinutes/1 -> Relational Operator2/2

== system APP_MyApplication/Model/APP_MyApplication_/DateTime/DateTimeAssemble/CheckIfInputIsValid/CheckIfMonthIsValid ==
  note: also check if month equals zero, to avoid error in 'CountDaysForCompleteMonths' Subsystem
  u8_Month : Inport  OutDataTypeStr=uint8
  u8_MaxMonth : Inport  Port=2  OutDataTypeStr=uint8
  u8_MinMonth : Inport  Port=3  OutDataTypeStr=uint8
  Logical Operator : Logic  AllPortsSameDT=off  OutDataTypeStr=boolean
  Relational Operator6 : RelationalOperator  Operator=<=  OutDataTypeStr=boolean  RndMeth=Nearest
  Relational Operator7 : RelationalOperator  OutDataTypeStr=boolean  RndMeth=Nearest
  bo_IsMonthValid : Outport  OutDataTypeStr=boolean
  wires:
  u8_MaxMonth/1 -> Relational Operator6/2
  u8_MinMonth/1 -> Relational Operator7/2
  u8_Month/1 -> Relational Operator7/1, Relational Operator6/1
  Relational Operator6/1 -> Logical Operator/1
  Relational Operator7/1 -> Logical Operator/2
  Logical Operator/1 -> bo_IsMonthValid/1

== system APP_MyApplication/Model/APP_MyApplication_/DateTime/DateTimeAssemble/CheckIfInputIsValid/CheckIfSecondsAreValid ==
  note: check if seconds data is valid
  u8_SecondsIn : Inport  OutDataTypeStr=uint8
  u8_MaxSeconds : Inport  Port=2  OutDataTypeStr=uint8
  Relational Operator : RelationalOperator  Operator=<=  OutDataTypeStr=boolean  RndMeth=Nearest
  bo_AreSecondsValid : Outport  OutDataTypeStr=boolean
  wires:
  Relational Operator/1 -> bo_AreSecondsValid/1
  u8_SecondsIn/1 -> Relational Operator/1
  u8_MaxSeconds/1 -> Relational Operator/2

== system APP_MyApplication/Model/APP_MyApplication_/DateTime/DateTimeAssemble/CheckIfInputIsValid/CheckIfYearIsValid ==
  note: check if year is greater than or equal to 1970
  note: check if year is less than or equal to 2099
  u16_YearIn : Inport  OutDataTypeStr=uint16
  u16_MinYear : Inport  Port=2  OutDataTypeStr=uint16
  u16_MaxYear : Inport  Port=3  OutDataTypeStr=uint16
  Relational Operator : RelationalOperator  OutDataTypeStr=boolean  RndMeth=Nearest
  Relational Operator1 : RelationalOperator  Operator=<=  OutDataTypeStr=boolean  RndMeth=Nearest
  bo_IsGreaterOrEqualMin : Outport  OutDataTypeStr=boolean
  bo_IsLessOrEqualMax : Outport  Port=2  OutDataTypeStr=boolean
  wires:
  u16_YearIn/1 -> Relational Operator1/1, Relational Operator/1
  u16_MinYear/1 -> Relational Operator/2
  u16_MaxYear/1 -> Relational Operator1/2
  Relational Operator/1 -> bo_IsGreaterOrEqualMin/1
  Relational Operator1/1 -> bo_IsLessOrEqualMax/1

== system APP_MyApplication/Model/APP_MyApplication_/DateTime/DateTimeAssemble/ConvertToDateTime/ConvertDaysToSeconds ==
  note: 86400 sec/d
  note: convert days to seconds
  u16_NrOfDays : Inport  OutDataTypeStr=uint16
  Constant : Constant  Value=86400  OutDataTypeStr=uint32
  Product : Product  OutDataTypeStr=uint32
  u32_SecFromDays : Outport  OutDataTypeStr=uint32
  wires:
  u16_NrOfDays/1 -> Product/1
  Constant/1 -> Product/2
  Product/1 -> u32_SecFromDays/1

== system APP_MyApplication/Model/APP_MyApplication_/DateTime/DateTimeAssemble/ConvertToDateTime/ConvertHoursToSeconds ==
  note: 3600 sec/h
  note: convert hours to seconds
  u8_Hours : Inport  OutDataTypeStr=uint8
  Constant1 : Constant  Value=3600  OutDataTypeStr=uint16
  Product1 : Product  OutDataTypeStr=uint32
  u32_SecFromHrs : Outport  OutDataTypeStr=uint32
  wires:
  u8_Hours/1 -> Product1/1
  Constant1/1 -> Product1/2
  Product1/1 -> u32_SecFromHrs/1

== system APP_MyApplication/Model/APP_MyApplication_/DateTime/DateTimeAssemble/ConvertToDateTime/ConvertMinutesToSeconds ==
  note: 60 sec/min
  note: convert minutes to seconds
  u8_Minutes : Inport  OutDataTypeStr=uint8
  Constant : Constant  Value=60  OutDataTypeStr=uint8
  Product : Product  OutDataTypeStr=uint16
  u16_SecFromMins : Outport  OutDataTypeStr=uint16
  wires:
  Product/1 -> u16_SecFromMins/1
  Constant/1 -> Product/2
  u8_Minutes/1 -> Product/1

== system APP_MyApplication/Model/APP_MyApplication_/DateTime/DateTimeAssemble/ConvertToNrOfDays/AddDays ==
  u8_Day : Inport  OutDataTypeStr=uint8
  Constant5 : Constant  OutDataTypeStr=uint8
  Subtract4 : Sum  Inputs=+-  OutDataTypeStr=uint8
  u8_CompleteDays : Outport  OutDataTypeStr=uint8
  wires:
  Constant5/1 -> Subtract4/2
  u8_Day/1 -> Subtract4/1
  Subtract4/1 -> u8_CompleteDays/1

== system APP_MyApplication/Model/APP_MyApplication_/DateTime/DateTimeAssemble/ConvertToNrOfDays/AddDaysForCompleteMonths ==
  note: add days for complete months
  u8_Month : Inport  OutDataTypeStr=uint8
  Add2 : Sum  OutDataTypeStr=uint16
  Constant1 : Constant  Value=[0 31 28 31 30 31 30 31 31 30 31 30]  OutDataTypeStr=uint8
  For Iterator : ForIterator  ResetStates=reset  IterationSource=external  IndexMode=Zero-based
  Selector : Selector  IndexMode=Zero-based  InputPortWidth=12  IndexOptions=Index vector (port)  Indices=[1 3]  OutputSizes=1
  Unit Delay1 : UnitDelay  SampleTime=-1
  u16_DaysForMonths : Outport  OutDataTypeStr=uint16
  wires:
  Constant1/1 -> Selector/1
  For Iterator/1 -> Selector/2
  u8_Month/1 -> For Iterator/1
  Selector/1 -> Add2/1
  Unit Delay1/1 -> Add2/2
  Add2/1 -> u16_DaysForMonths/1, Unit Delay1/1

== system APP_MyApplication/Model/APP_MyApplication_/DateTime/DateTimeAssemble/ConvertToNrOfDays/AddDaysForCompleteYears ==
  note: count leap days since 1970
  note: add days for complete years
  u16_Year : Inport  OutDataTypeStr=uint16
  Add : Sum  Inputs=+-  OutDataTypeStr=uint16
  Add1 : Sum  OutDataTypeStr=uint16
  Constant : Constant  Value=1970  OutDataTypeStr=uint16
  Constant1 : Constant  Value=365  OutDataTypeStr=uint16
  Constant2 : Constant  Value=1968  OutDataTypeStr=uint16
  Constant3 : Constant  Value=4  OutDataTypeStr=uint16
  Divide : Product  Inputs=*/  OutDataTypeStr=uint16
  Product : Product  OutDataTypeStr=uint16
  Subtract : Sum  Inputs=+-  OutDataTypeStr=uint16
  u16_DaysForYears : Outport  OutDataTypeStr=uint16
  wires:
  u16_Year/1 -> Subtract/1, Add/1
  Constant/1 -> Add/2
  Add/1 -> Product/1
  Constant1/1 -> Product/2
  Constant2/1 -> Subtract/2
  Subtract/1 -> Divide/1
  Constant3/1 -> Divide/2
  Product/1 -> Add1/1
  Divide/1 -> Add1/2
  Add1/1 -> u16_DaysForYears/1

== system APP_MyApplication/Model/APP_MyApplication_/DateTime/DateTimeAssemble/ConvertToNrOfDays/CheckIfDateInLeapYearBeforeMarch ==
  note: check if the date is in leap year and before the leap day
  u8_Month : Inport  OutDataTypeStr=uint8
  u16_Year : Inport  Port=2  OutDataTypeStr=uint16
  Constant2 : Constant  Value=1968  OutDataTypeStr=uint16
  Constant3 : Constant  Value=4  OutDataTypeStr=uint16
  Constant6 : Constant  Value=0  OutDataTypeStr=uint16
  Constant7 : Constant  Value=2  OutDataTypeStr=uint8
  Logical Operator : Logic  AllPortsSameDT=off  OutDataTypeStr=boolean
  Math Function : Math  Operator=rem  OutputSignalType=real  SaturateOnIntegerOverflow=on
  Relational Operator1 : RelationalOperator  Operator===  OutDataTypeStr=boolean  RndMeth=Nearest  InputSameDT=on
  Relational Operator3 : RelationalOperator  Operator=<=  OutDataTypeStr=boolean  RndMeth=Nearest
  Subtract : Sum  Inputs=+-  OutDataTypeStr=uint16
  bo_MinusOne : Outport  OutDataTypeStr=boolean
  wires:
  u16_Year/1 -> Subtract/1
  Constant2/1 -> Subtract/2
  Subtract/1 -> Math Function/1
  Constant3/1 -> Math Function/2
  Math Function/1 -> Relational Operator1/1
  Constant6/1 -> Relational Operator1/2
  Constant7/1 -> Relational Operator3/2
  Relational Operator1/1 -> Logical Operator/1
  Relational Operator3/1 -> Logical Operator/2
  u8_Month/1 -> Relational Operator3/1
  Logical Operator/1 -> bo_MinusOne/1

== system APP_MyApplication/Model/APP_MyApplication_/DateTime/DateTimeAssemble1/CheckIfInputIsValid/CheckIfDayIsValid ==
  note: Index correction
  note: days per month
  note: check if day data is valid
  u8_DayIn : Inport  OutDataTypeStr=uint8
  u8_MonthIn : Inport  Port=2  OutDataTypeStr=uint8
  u16_YearIn : Inport  Port=3  OutDataTypeStr=uint16
  u8_MinDay : Inport  Port=4  OutDataTypeStr=uint8
  bo_IsMonthValid : Inport  Port=5  OutDataTypeStr=boolean
  CheckIfFebruaryOfLeapYear : Subsystem
  Constant1 : Constant  OutDataTypeStr=uint8
  Constant2 : Constant  Value=[31 28 31 30 31 30 31 31 30 31 30 31]  OutDataTypeStr=uint8
  Constant20 : Constant  OutDataTypeStr=uint8
  Logical Operator1 : Logic  AllPortsSameDT=off  OutDataTypeStr=boolean
  Logical Operator3 : Logic  Operator=OR  AllPortsSameDT=off  OutDataTypeStr=boolean
  Relational Operator4 : RelationalOperator  Operator=<=  OutDataTypeStr=boolean  RndMeth=Nearest
  Relational Operator8 : RelationalOperator  OutDataTypeStr=boolean  RndMeth=Nearest
  Selector : Selector  IndexMode=Zero-based  InputPortWidth=12  IndexOptions=Index vector (port)  Indices=[1 3]  OutputSizes=1
  Subtract : Sum  Inputs=+-  OutDataTypeStr=uint8
      settings: AttributesFormatString=Saturate: %<SaturateOnIntegerOverflow>
  Switch2 : Switch  Criteria=u2 > Threshold  OutDataTypeStr=uint8
  bo_IsDayValid : Outport  OutDataTypeStr=boolean
  wires:
  u16_YearIn/1 -> CheckIfFebruaryOfLeapYear/3(u16_YearIn)
  Constant2/1 -> Selector/1
  u8_MonthIn/1 -> CheckIfFebruaryOfLeapYear/2(u8_MonthIn), Switch2/1
  Selector/1 -> Relational Operator4/2
  Relational Operator4/1 -> Logical Operator3/1
  Relational Operator8/1 -> Logical Operator1/1
  Constant20/1 -> Switch2/3
  Logical Operator3/1 -> Logical Operator1/2
  Logical Operator1/1 -> bo_IsDayValid/1
  u8_DayIn/1 -> Relational Operator8/1, Relational Operator4/1, CheckIfFebruaryOfLeapYear/1(u8_DayIn)
  CheckIfFebruaryOfLeapYear/1(bo_IsFebrauryOfLeapYear) -> Logical Operator3/2
  u8_MinDay/1 -> Relational Operator8/2
  bo_IsMonthValid/1 -> Switch2/2
  Switch2/1 -> Subtract/1
  Subtract/1 -> Selector/2
  Constant1/1 -> Subtract/2

== system APP_MyApplication/Model/APP_MyApplication_/DateTime/DateTimeAssemble1/CheckIfInputIsValid/CheckIfHoursAreValid ==
  note: check if hours data is valid
  u8_HoursIn : Inport  OutDataTypeStr=uint8
  u8_MaxHours : Inport  Port=2  OutDataTypeStr=uint8
  Relational Operator3 : RelationalOperator  Operator=<=  OutDataTypeStr=boolean  RndMeth=Nearest
  bo_AreHoursValid : Outport  OutDataTypeStr=boolean
  wires:
  Relational Operator3/1 -> bo_AreHoursValid/1
  u8_HoursIn/1 -> Relational Operator3/1
  u8_MaxHours/1 -> Relational Operator3/2

== system APP_MyApplication/Model/APP_MyApplication_/DateTime/DateTimeAssemble1/CheckIfInputIsValid/CheckIfMinutesAreValid ==
  note: check if minutes data is valid
  u8_MinutesIn : Inport  OutDataTypeStr=uint8
  u8_MaxMinutes : Inport  Port=2  OutDataTypeStr=uint8
  Relational Operator2 : RelationalOperator  Operator=<=  OutDataTypeStr=boolean  RndMeth=Nearest
  bo_AreMinutesValid : Outport  OutDataTypeStr=boolean
  wires:
  Relational Operator2/1 -> bo_AreMinutesValid/1
  u8_MinutesIn/1 -> Relational Operator2/1
  u8_MaxMinutes/1 -> Relational Operator2/2

== system APP_MyApplication/Model/APP_MyApplication_/DateTime/DateTimeAssemble1/CheckIfInputIsValid/CheckIfMonthIsValid ==
  note: also check if month equals zero, to avoid error in 'CountDaysForCompleteMonths' Subsystem
  u8_Month : Inport  OutDataTypeStr=uint8
  u8_MaxMonth : Inport  Port=2  OutDataTypeStr=uint8
  u8_MinMonth : Inport  Port=3  OutDataTypeStr=uint8
  Logical Operator : Logic  AllPortsSameDT=off  OutDataTypeStr=boolean
  Relational Operator6 : RelationalOperator  Operator=<=  OutDataTypeStr=boolean  RndMeth=Nearest
  Relational Operator7 : RelationalOperator  OutDataTypeStr=boolean  RndMeth=Nearest
  bo_IsMonthValid : Outport  OutDataTypeStr=boolean
  wires:
  u8_MaxMonth/1 -> Relational Operator6/2
  u8_MinMonth/1 -> Relational Operator7/2
  u8_Month/1 -> Relational Operator7/1, Relational Operator6/1
  Relational Operator6/1 -> Logical Operator/1
  Relational Operator7/1 -> Logical Operator/2
  Logical Operator/1 -> bo_IsMonthValid/1

== system APP_MyApplication/Model/APP_MyApplication_/DateTime/DateTimeAssemble1/CheckIfInputIsValid/CheckIfSecondsAreValid ==
  note: check if seconds data is valid
  u8_SecondsIn : Inport  OutDataTypeStr=uint8
  u8_MaxSeconds : Inport  Port=2  OutDataTypeStr=uint8
  Relational Operator : RelationalOperator  Operator=<=  OutDataTypeStr=boolean  RndMeth=Nearest
  bo_AreSecondsValid : Outport  OutDataTypeStr=boolean
  wires:
  Relational Operator/1 -> bo_AreSecondsValid/1
  u8_SecondsIn/1 -> Relational Operator/1
  u8_MaxSeconds/1 -> Relational Operator/2

== system APP_MyApplication/Model/APP_MyApplication_/DateTime/DateTimeAssemble1/CheckIfInputIsValid/CheckIfYearIsValid ==
  note: check if year is greater than or equal to 1970
  note: check if year is less than or equal to 2099
  u16_YearIn : Inport  OutDataTypeStr=uint16
  u16_MinYear : Inport  Port=2  OutDataTypeStr=uint16
  u16_MaxYear : Inport  Port=3  OutDataTypeStr=uint16
  Relational Operator : RelationalOperator  OutDataTypeStr=boolean  RndMeth=Nearest
  Relational Operator1 : RelationalOperator  Operator=<=  OutDataTypeStr=boolean  RndMeth=Nearest
  bo_IsGreaterOrEqualMin : Outport  OutDataTypeStr=boolean
  bo_IsLessOrEqualMax : Outport  Port=2  OutDataTypeStr=boolean
  wires:
  u16_YearIn/1 -> Relational Operator1/1, Relational Operator/1
  u16_MinYear/1 -> Relational Operator/2
  u16_MaxYear/1 -> Relational Operator1/2
  Relational Operator/1 -> bo_IsGreaterOrEqualMin/1
  Relational Operator1/1 -> bo_IsLessOrEqualMax/1

== system APP_MyApplication/Model/APP_MyApplication_/DateTime/DateTimeAssemble1/ConvertToDateTime/ConvertDaysToSeconds ==
  note: 86400 sec/d
  note: convert days to seconds
  u16_NrOfDays : Inport  OutDataTypeStr=uint16
  Constant : Constant  Value=86400  OutDataTypeStr=uint32
  Product : Product  OutDataTypeStr=uint32
  u32_SecFromDays : Outport  OutDataTypeStr=uint32
  wires:
  u16_NrOfDays/1 -> Product/1
  Constant/1 -> Product/2
  Product/1 -> u32_SecFromDays/1

== system APP_MyApplication/Model/APP_MyApplication_/DateTime/DateTimeAssemble1/ConvertToDateTime/ConvertHoursToSeconds ==
  note: 3600 sec/h
  note: convert hours to seconds
  u8_Hours : Inport  OutDataTypeStr=uint8
  Constant1 : Constant  Value=3600  OutDataTypeStr=uint16
  Product1 : Product  OutDataTypeStr=uint32
  u32_SecFromHrs : Outport  OutDataTypeStr=uint32
  wires:
  u8_Hours/1 -> Product1/1
  Constant1/1 -> Product1/2
  Product1/1 -> u32_SecFromHrs/1

== system APP_MyApplication/Model/APP_MyApplication_/DateTime/DateTimeAssemble1/ConvertToDateTime/ConvertMinutesToSeconds ==
  note: 60 sec/min
  note: convert minutes to seconds
  u8_Minutes : Inport  OutDataTypeStr=uint8
  Constant : Constant  Value=60  OutDataTypeStr=uint8
  Product : Product  OutDataTypeStr=uint16
  u16_SecFromMins : Outport  OutDataTypeStr=uint16
  wires:
  Product/1 -> u16_SecFromMins/1
  Constant/1 -> Product/2
  u8_Minutes/1 -> Product/1

== system APP_MyApplication/Model/APP_MyApplication_/DateTime/DateTimeAssemble1/ConvertToNrOfDays/AddDays ==
  u8_Day : Inport  OutDataTypeStr=uint8
  Constant5 : Constant  OutDataTypeStr=uint8
  Subtract4 : Sum  Inputs=+-  OutDataTypeStr=uint8
  u8_CompleteDays : Outport  OutDataTypeStr=uint8
  wires:
  Constant5/1 -> Subtract4/2
  u8_Day/1 -> Subtract4/1
  Subtract4/1 -> u8_CompleteDays/1

== system APP_MyApplication/Model/APP_MyApplication_/DateTime/DateTimeAssemble1/ConvertToNrOfDays/AddDaysForCompleteMonths ==
  note: add days for complete months
  u8_Month : Inport  OutDataTypeStr=uint8
  Add2 : Sum  OutDataTypeStr=uint16
  Constant1 : Constant  Value=[0 31 28 31 30 31 30 31 31 30 31 30]  OutDataTypeStr=uint8
  For Iterator : ForIterator  ResetStates=reset  IterationSource=external  IndexMode=Zero-based
  Selector : Selector  IndexMode=Zero-based  InputPortWidth=12  IndexOptions=Index vector (port)  Indices=[1 3]  OutputSizes=1
  Unit Delay1 : UnitDelay  SampleTime=-1
  u16_DaysForMonths : Outport  OutDataTypeStr=uint16
  wires:
  Constant1/1 -> Selector/1
  For Iterator/1 -> Selector/2
  u8_Month/1 -> For Iterator/1
  Selector/1 -> Add2/1
  Unit Delay1/1 -> Add2/2
  Add2/1 -> u16_DaysForMonths/1, Unit Delay1/1
